simulink model "nasheq_model"  (R2023a)
settings: Solver=VariableStepAuto  StartTime=0.0  StopTime=6  RelTol=1e-3
values from neighbouring files (symbols this model uses):
  BESS2 =     [state_space.mat]    (also in state_space_and_controllers.mat)
  BESS3 =     [state_space.mat]    (also in state_space_and_controllers.mat)
  BESS6 =     [state_space.mat]    (also in state_space_and_controllers.mat)
  Grid =     [state_space.mat]    (also in state_space_and_controllers.mat)
  Load =     [state_space.mat]    (also in state_space_and_controllers.mat)
  PV1 =     [state_space.mat]    (also in state_space_and_controllers.mat)
  PV4 =     [state_space.mat]    (also in state_space_and_controllers.mat)
  PV5 =     [state_space.mat]    (also in state_space_and_controllers.mat)
  Ts = 0.0001    [cost_analysis.m]    (also in simulation_run.m)
libraries: slpidlib x6, spspowerguiLib x1
settings Model: Creator=paul  LastModifiedBy=paul
settings DataIOCC: Refine=4

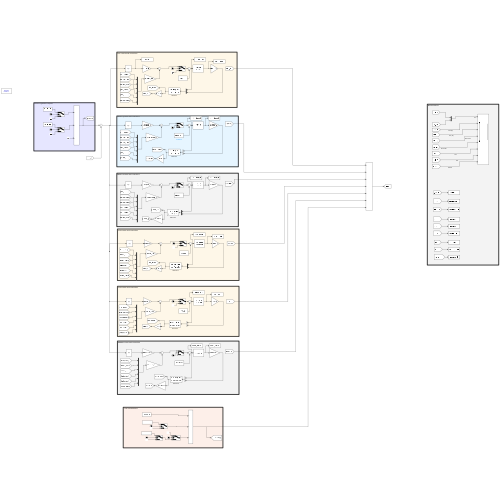
[thumbnail: Simulink's stored preview of the top-level diagram]
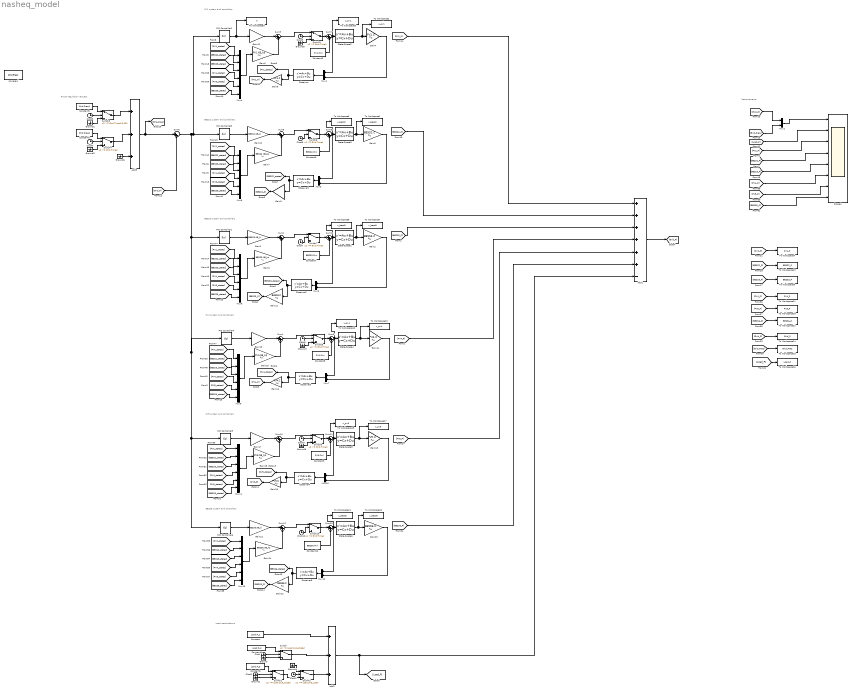
== system nasheq_model ==
  note: BESS2 system and controllers
  note: Measurements
  note: PV1 system and controllers
  note: Load perturbations
  note: Power regulation request
  note: BESS3 system and controllers
  note: PV4 system and controllers
  note: PV5 system and controllers
  note: BESS6 system and controllers
  Add1 : Sum  Inputs=++++++-
  Add2 : Sum  Inputs=+++
  Add3 : Sum  Inputs=+++
  Clock{,1..10} (11 alike) : Clock
  Constant : Constant  Value=Load.P_1
  Constant1 : Constant  Value=Load.P_2
  Constant10 : Constant  Value=BESS6.Pini
  Constant2 : Constant  Value=Load.P_3
  Constant3 : Constant  Value=Grid.Preq1
  Constant4 : Constant  Value=Grid.Preq2
  Constant5 : Constant  Value=PV1.Pini
  Constant6 : Constant  Value=BESS2.Pini
  Constant7 : Constant  Value=BESS3.Pini
  Constant8 : Constant  Value=PV4.Pini
  Constant9 : Constant  Value=PV5.Pini
  Gain1 : Gain  Gain=BESS3.NE_ki
  Gain10 : Gain  Gain=BESS2.NE_ki
  Gain11 : Gain  Gain=PV1.NE_ki
  Gain12 : Gain  Gain=BESS3.C  Multiplication=Matrix(K*u)
  Gain13 : Gain  Gain=PV4.NE_ki
  Gain14 : Gain  Gain=PV4.C  Multiplication=Matrix(K*u)
  Gain15 : Gain  Gain=PV4.NE_kp  Multiplication=Matrix(K*u)
  Gain16 : Gain  Gain=PV4.C  Multiplication=Matrix(K*u)
  Gain17 : Gain  Gain=PV5.NE_ki
  Gain18 : Gain  Gain=PV5.C  Multiplication=Matrix(K*u)
  Gain19 : Gain  Gain=PV5.NE_kp  Multiplication=Matrix(K*u)
  Gain2 : Gain  Gain=BESS3.C  Multiplication=Matrix(K*u)
  Gain20 : Gain  Gain=PV5.C  Multiplication=Matrix(K*u)
  Gain21 : Gain  Gain=BESS6.NE_ki
  Gain22 : Gain  Gain=BESS6.C  Multiplication=Matrix(K*u)
  Gain23 : Gain  Gain=BESS6.C  Multiplication=Matrix(K*u)
  Gain24 : Gain  Gain=BESS6.NE_kp  Multiplication=Matrix(K*u)
  Gain3 : Gain  Gain=BESS3.NE_kp  Multiplication=Matrix(K*u)
  Gain4 : Gain  Gain=PV1.C  Multiplication=Matrix(K*u)
  Gain5 : Gain  Gain=BESS2.C  Multiplication=Matrix(K*u)
  Gain6 : Gain  Gain=PV1.NE_kp  Multiplication=Matrix(K*u)
  Gain7 : Gain  Gain=BESS2.NE_kp  Multiplication=Matrix(K*u)
  Gain8 : Gain  Gain=PV1.C  Multiplication=Matrix(K*u)
  Gain9 : Gain  Gain=BESS2.C  Multiplication=Matrix(K*u)
  Ground{,1..8} (9 alike) : Ground
  Mux{1..3,6..7,10,12} (7 alike) : Mux  Inputs=2
  Mux{4..5,8..9,11,13} (6 alike) : Mux  Inputs=6
  Observer : StateSpace  A=PV1.kf_As  B=PV1.kf_Bs  C=PV1.kf_Cs  D=PV1.kf_Ds  InitialCondition=0
  Observer1 : StateSpace  A=BESS2.kf_As  B=BESS2.kf_Bs  C=BESS2.kf_Cs  D=BESS2.kf_Ds  InitialCondition=0
  Observer2 : StateSpace  A=BESS3.kf_As  B=BESS3.kf_Bs  C=BESS3.kf_Cs  D=BESS3.kf_Ds  InitialCondition=0
  Observer3 : StateSpace  A=PV4.kf_As  B=PV4.kf_Bs  C=PV4.kf_Cs  D=PV4.kf_Ds  InitialCondition=0
  Observer4 : StateSpace  A=PV5.kf_As  B=PV5.kf_Bs  C=PV5.kf_Cs  D=PV5.kf_Ds  InitialCondition=0
  Observer5 : StateSpace  A=BESS6.kf_As  B=BESS6.kf_Bs  C=BESS6.kf_Cs  D=BESS6.kf_Ds  InitialCondition=0
  PID Controller{1..6} (6 alike) : slpidlib/PID Controller  Controller=I  Form=Parallel  TimeDomain=Continuous-time  UseExternalTs=off  SampleTime=-1  IntegratorMethod=Forward Euler  FilterMethod=Forward Euler  ControllerParametersSource=internal  P=1  I=1  UseKiTs=off  D=0  N=100  UseFilter=on  TunerSelectOption=Transfer Function Based (PID Tuner App)  InitialConditionSource=internal  InitialConditionForIntegrator=0  InitialConditionForFilter=0  DifferentiatorICPrevScaledInput=0  ExternalReset=none  TrackingMode=off  Kt=1  LimitOutput=off  SatLimitsSource=internal  UpperSaturationLimit=inf  LowerSaturationLimit=-inf  LinearizeAsGain=on  AntiWindupMode=none  Kb=1  LimitIntegrator=off  UpperIntegratorSaturationLimit=inf  LowerIntegratorSaturationLimit=-inf  POutMin=[]  POutMax=[]  IOutMin=[]  IOutMax=[]  DOutMin=[]  DOutMax=[]  NOutMin=[]  NOutMax=[]  SumOutMin=[]  SumOutMax=[]  SaturationOutMin=[]  SaturationOutMax=[]  PParamMin=[]  PParamMax=[]  IParamMin=[]  IParamMax=[]  DParamMin=[]  DParamMax=[]  NParamMin=[]  NParamMax=[]  KbParamMin=[]  KbParamMax=[]  KtParamMin=[]  KtParamMax=[]  KbOutMin=[]  KbOutMax=[]  KtOutMin=[]  KtOutMax=[]  IntegratorOutMin=[]  IntegratorOutMax=[]  FilterOutMin=[]  FilterOutMax=[]  SumI1OutMin=[]  SumI1OutMax=[]  SumI2OutMin=[]  SumI2OutMax=[]  SumI3OutMin=[]  SumI3OutMax=[]  SumI4OutMin=[]  SumI4OutMax=[]  SumDOutMin=[]  SumDOutMax=[]  DifferentiatorOutMin=[]  DifferentiatorOutMax=[]  FilterDiffOutCoefMin=[]  FilterDiffOutCoefMax=[]  ReciprocalOutMin=[]  ReciprocalOutMax=[]  SumDenOutMin=[]  SumDenOutMax=[]  SumNumOutMin=[]  SumNumOutMax=[]  DivideOutMin=[]  DivideOutMax=[]  UdiffTsProdOutMin=[]  UdiffTsProdOutMax=[]  NTsProdOutMin=[]  NTsProdOutMax=[]  UintegralTsProdOutMin=[]  UintegralTsProdOutMax=[]  UngainTsProdOutMin=[]  UngainTsProdOutMax=[]  ClampingZeroOutDataTypeStr=Inherit: Inherit via back propagation  ClampingZeroOutMin=[]  ClampingZeroOutMax=[]  FilterDenConstantOutDataTypeStr=Inherit: Inherit via back propagation  FilterDenConstantOutMin=[]  FilterDenConstantOutMax=[]  PCopyOutDataTypeStr=Inherit: Inherit via back propagation  PCopyOutMin=[]  PCopyOutMax=[]  NCopyOutDataTypeStr=Inherit: Inherit via back propagation  NCopyOutMin=[]  NCopyOutMax=[]  IntegratorContinuousStateAttributes=''  IntegratorStateMustResolveToSignalObject=off  IntegratorRTWStateStorageClass=Auto  FilterContinuousStateAttributes=''  FilterStateMustResolveToSignalObject=off  FilterRTWStateStorageClass=Auto  ParallelPVariant=Disabled  IdealPVariant=Disabled  IVariant=InternalParameters  DVariant=Disabled  IntegratorVariant=Continuous  SatVariant=Disabled  AWVariant=Passthrough  PCopyVariant=Disabled  TRVariant=Disabled  FdbkBlocksVariant=Forward  IdealPFdbkVariant=Disabled  SatFdbkVariant=Disabled  DerivativeFilterVariant=Disabled  NVariant=Disabled  NCopyVariant=Disabled_SignalSpec  FilterICVariant=Disabled  IntegratorICVariant=InternalICs  ExternalResetVariant=Disabled  TRSumVariant=Passthrough  SumFdbkVariant=Disabled  SumVariant=Passthrough_I  TsampFilterVariant=InternalTs  TsampNgainVariant=Passthrough  TsampIntegralVariant=Disabled_SignalSpec  ExternalSaturationOutDataTypeStr=Inherit: Same as second input
  Scope1 : Scope  NumInputPorts=8
  State-Space1 : StateSpace  A=BESS3.A  B=BESS3.B  C=eye(2,2)  D=zeros(2,1)  InitialCondition=0
  State-Space2 : StateSpace  A=PV1.A  B=PV1.B  C=eye(2,2)  D=zeros(2,1)  InitialCondition=0
  State-Space3 : StateSpace  A=BESS2.A  B=BESS2.B  C=eye(2,2)  D=zeros(2,1)  InitialCondition=0
  State-Space4 : StateSpace  A=PV4.A  B=PV4.B  C=eye(2,2)  D=zeros(2,1)  InitialCondition=0
  State-Space5 : StateSpace  A=PV5.A  B=PV5.B  C=eye(2,2)  D=zeros(2,1)  InitialCondition=0
  State-Space6 : StateSpace  A=BESS6.A  B=BESS6.B  C=eye(2,2)  D=zeros(2,1)  InitialCondition=0
  Sum{1..5,7..13} (12 alike) : Sum  Inputs=|++
  Sum6 : Sum  Inputs=|+-
  Switch : Switch  Threshold=Load.sw2_closed  SaturateOnIntegerOverflow=off  InputSameDT=off
  Switch1 : Switch  Threshold=Load.sw3_closed  SaturateOnIntegerOverflow=off  InputSameDT=off
  Switch{5..10} (6 alike) : Switch  Threshold=Grid.Time1  SaturateOnIntegerOverflow=off  InputSameDT=off
  Switch2 : Switch  Threshold=Load.sw3_open  SaturateOnIntegerOverflow=off  InputSameDT=off
  Switch3 : Switch  Threshold=Grid.Time1-0.001  SaturateOnIntegerOverflow=off  InputSameDT=off
  Switch4 : Switch  Threshold=Grid.Time2  SaturateOnIntegerOverflow=off  InputSameDT=off
  To Workspace1 : ToWorkspace  VariableName=x_bess2  SaveFormat=Timeseries  SampleTime=Ts
  To Workspace10 : ToWorkspace  VariableName=x_pv4  SaveFormat=Timeseries  SampleTime=Ts
  To Workspace11 : ToWorkspace  VariableName=PV4_P  SaveFormat=Timeseries  SampleTime=Ts
  To Workspace12 : ToWorkspace  VariableName=u_pv4  SaveFormat=Timeseries  SampleTime=Ts
  To Workspace13 : ToWorkspace  VariableName=BESS2_P  SaveFormat=Timeseries  SampleTime=Ts
  To Workspace14 : ToWorkspace  VariableName=Grid_P  SaveFormat=Timeseries  SampleTime=Ts
  To Workspace15 : ToWorkspace  VariableName=Grid_Preq  SaveFormat=Timeseries  SampleTime=Ts
  To Workspace16 : ToWorkspace  VariableName=Load_P  SaveFormat=Timeseries  SampleTime=Ts
  To Workspace17 : ToWorkspace  VariableName=x_pv5  SaveFormat=Timeseries  SampleTime=Ts
  To Workspace18 : ToWorkspace  VariableName=PV5_P  SaveFormat=Timeseries  SampleTime=Ts
  To Workspace19 : ToWorkspace  VariableName=u_pv5  SaveFormat=Timeseries  SampleTime=Ts
  To Workspace2 : ToWorkspace  VariableName=x_pv1  SaveFormat=Timeseries  SampleTime=Ts
  To Workspace20 : ToWorkspace  VariableName=x_bess6  SaveFormat=Timeseries  SampleTime=Ts
  To Workspace21 : ToWorkspace  VariableName=u_bess6  SaveFormat=Timeseries  SampleTime=Ts
  To Workspace22 : ToWorkspace  VariableName=BESS6_P  SaveFormat=Timeseries  SampleTime=Ts
  To Workspace3 : ToWorkspace  VariableName=w  SaveFormat=Timeseries  SampleTime=Ts
  To Workspace4 : ToWorkspace  VariableName=PV1_P  SaveFormat=Timeseries  SampleTime=Ts
  To Workspace5 : ToWorkspace  VariableName=u_pv1  SaveFormat=Timeseries  SampleTime=Ts
  To Workspace6 : ToWorkspace  VariableName=u_bess2  SaveFormat=Timeseries  SampleTime=Ts
  To Workspace7 : ToWorkspace  VariableName=x_bess3  SaveFormat=Timeseries  SampleTime=Ts
  To Workspace8 : ToWorkspace  VariableName=u_bess3  SaveFormat=Timeseries  SampleTime=Ts
  To Workspace9 : ToWorkspace  VariableName=BESS3_P  SaveFormat=Timeseries  SampleTime=Ts
  powergui : spspowerguiLib/powergui  Priority=1  SimulationMode=Discrete  SampleTime=Ts  frequency=60  Iterations=50  frequencyindice=60  Pbase=100e6  ErrMax=1e-4  UnitsV=kV  UnitsW=MW  buscounter=0  FunctionMessages=off  echomessages=off  EnableUseOfTLC=off  CurrentSourceSwitches=off  DisableSnubberDevices=off  DisableRonSwitches=off  DisableVfSwitches=off  DisplayEquations=off  AutomaticDiscreteSolvers=off  SolverType=Tustin/Backward Euler (TBE)  Interpol=off  ExternalGateDelay=off  methode=off  Ts=100  x0status=blocks  SPID=on  SwTol=0  HookPort=off  NonlinearTolerance=1e-4  nMaxIteration=100  ContinueOnMaxIteration=off  RestoreLinks=warning  ResistiveCurrentMeasurement=off  Frange=[0:2:500]  Ylog=off  Xlog=on  ShowGrid=off  save=off  variable=ZData  structure=0  ZoomFFT=off  StartTime=0.0  cycles=1  DisplayStyle=1  fundamental=60  FreqAxis=off  MaxFrequency=1000  frequencyindicesteady=1  RmsSteady=1  display=off
  wires:
  Mux1/1 -> Observer/1
  Add1/1 -> [Grid_P]
  [BESS2_P] -> Scope1/4  "BESS2 (W)"
  Sum3/1 -> Switch5/1
  PID Controller3/1 -> Gain10/1
  Mux4/1 -> Gain6/1
  State-Space2/1 -> To Workspace2/1, Gain4/1
  Gain6/1 -> Sum3/2
  State-Space3/1 -> To Workspace1/1, Gain5/1
  Gain7/1 -> Sum5/2
  PID Controller2/1 -> To Workspace3/1, Gain11/1
  [PV1_P] -> Scope1/3  "PV1 (W)"
  Gain5/1 -> Mux3/2
  Mux3/1 -> Observer1/1
  Sum5/1 -> Switch6/1
  [PV1_states] -> Mux4/1
  Observer/1 -> Gain8/1, [PV1_states]
  [BESS2_states] -> Mux4/2
  Observer1/1 -> Gain9/1, [BESS2_states]
  Constant/1 -> Add2/1
  Constant1/1 -> Switch/1
  Clock/1 -> Switch/2
  Ground/1 -> Switch/3
  Switch/1 -> Add2/2
  [Load_P] -> Scope1/2  "Load (W)"
  [Grid_P] -> Sum6/2
  Ground1/1 -> Switch1/3
  Constant2/1 -> Switch1/1
  Clock1/1 -> Switch1/2
  Switch2/1 -> Add2/3
  Clock2/1 -> Switch2/2
  Switch1/1 -> Switch2/3
  Constant3/1 -> Switch3/1
  Clock3/1 -> Switch3/2
  Ground2/1 -> Switch3/3
  Switch3/1 -> Add3/1
  Add3/1 -> [Grid_Preq], Sum6/1
  Clock4/1 -> Switch4/2
  Constant4/1 -> Switch4/1
  Ground3/1 -> Switch4/3
  Switch4/1 -> Add3/2
  [Grid_P] -> Mux2/1
  Mux2/1 -> Scope1/1  "Grid"
  [Grid_Preq] -> Mux2/2
  Ground4/1 -> Switch2/1
  Constant5/1 -> Sum7/2
  Sum7/1 -> To Workspace5/1, Mux1/1, State-Space2/1
  Constant6/1 -> Sum8/2
  Sum8/1 -> Mux3/1, To Workspace6/1, State-Space3/1
  Switch5/1 -> Sum7/1
  Clock5/1 -> Switch5/2
  Switch6/1 -> Sum8/1
  Clock6/1 -> Switch6/2
  Ground5/1 -> Switch5/3
  Ground6/1 -> Add3/3
  Gain4/1 -> Mux1/2
  Add2/1 -> [Load_P], Add1/7
  Gain8/1 -> [PV1_P]
  [PV1_P] -> Add1/1
  Gain9/1 -> [BESS2_P]
  [BESS2_P] -> Add1/2
  Gain10/1 -> Sum5/1
  Gain11/1 -> Sum3/1
  [Grid_Preq] -> To Workspace15/1
  [Grid_P] -> To Workspace14/1
  [BESS2_P] -> To Workspace13/1
  [PV1_P] -> To Workspace4/1
  [Load_P] -> To Workspace16/1
  Sum2/1 -> Mux6/1, To Workspace8/1, State-Space1/1
  Gain3/1 -> Sum1/2
  Clock7/1 -> Switch7/2
  State-Space1/1 -> To Workspace7/1, Gain2/1
  Sum1/1 -> Switch7/1
  Constant7/1 -> Sum2/2
  Switch7/1 -> Sum2/1
  Gain2/1 -> Mux6/2
  Gain1/1 -> Sum1/1
  PID Controller1/1 -> Gain1/1
  Observer2/1 -> Gain12/1, [BESS3_states]
  [BESS3_P] -> Add1/3
  Mux6/1 -> Observer2/1
  Gain12/1 -> [BESS3_P]
  [BESS3_P] -> Scope1/5  "BESS3 (W)"
  [BESS3_P] -> To Workspace9/1
  [BESS3_states] -> Mux4/3
  Mux7/1 -> Observer3/1
  Ground7/1 -> Switch8/3
  Clock8/1 -> Switch8/2
  Sum4/1 -> Switch8/1
  Gain16/1 -> [PV4_P]
  [PV4_P] -> Add1/4
  Observer3/1 -> Gain16/1, [PV4_states]
  Sum9/1 -> To Workspace12/1, Mux7/1, State-Space4/1
  Switch8/1 -> Sum9/1
  Gain15/1 -> Sum4/2
  Gain13/1 -> Sum4/1
  Gain14/1 -> Mux7/2
  Constant8/1 -> Sum9/2
  State-Space4/1 -> To Workspace10/1, Gain14/1
  PID Controller4/1 -> Gain13/1
  Mux10/1 -> Observer4/1
  Ground8/1 -> Switch9/3
  Clock9/1 -> Switch9/2
  Sum10/1 -> Switch9/1
  Gain20/1 -> [PV5_P]
  [PV5_P] -> Add1/5
  Observer4/1 -> Gain20/1, [PV5_states]
  Sum11/1 -> To Workspace19/1, Mux10/1, State-Space5/1
  Switch9/1 -> Sum11/1
  Gain19/1 -> Sum10/2
  Gain17/1 -> Sum10/1
  Gain18/1 -> Mux10/2
  Constant9/1 -> Sum11/2
  State-Space5/1 -> To Workspace17/1, Gain18/1
  PID Controller5/1 -> Gain17/1
  Constant10/1 -> Sum13/2
  Gain22/1 -> [BESS6_P]
  Sum13/1 -> Mux12/1, To Workspace21/1, State-Space6/1
  Observer5/1 -> Gain22/1, [BESS6_states]
  Gain23/1 -> Mux12/2
  [BESS6_P] -> Add1/6
  Gain21/1 -> Sum12/1
  Clock10/1 -> Switch10/2
  Switch10/1 -> Sum13/1
  State-Space6/1 -> To Workspace20/1, Gain23/1
  Sum12/1 -> Switch10/1
  Sum6/1 -> PID Controller4/1, PID Controller6/1, PID Controller5/1, PID Controller1/1, PID Controller2/1, PID Controller3/1
  Gain24/1 -> Sum12/2
  PID Controller6/1 -> Gain21/1
  Mux12/1 -> Observer5/1
  [PV4_states] -> Mux4/4
  [PV5_states] -> Mux4/5
  [BESS6_states] -> Mux4/6
  [BESS6_states] -> Mux5/6
  [PV4_states] -> Mux5/4
  Mux5/1 -> Gain7/1
  [PV5_states] -> Mux5/5
  [BESS2_states] -> Mux5/2
  [BESS3_states] -> Mux5/3
  [PV1_states] -> Mux5/1
  [PV1_states] -> Mux8/1
  [BESS6_states] -> Mux8/6
  [BESS3_states] -> Mux8/3
  [PV5_states] -> Mux8/5
  [BESS2_states] -> Mux8/2
  [PV4_states] -> Mux8/4
  Mux8/1 -> Gain3/1
  [PV5_states] -> Mux9/5
  [PV4_states] -> Mux9/4
  Mux9/1 -> Gain15/1
  [BESS6_states] -> Mux9/6
  [BESS2_states] -> Mux9/2
  [PV1_states] -> Mux9/1
  [BESS3_states] -> Mux9/3
  [BESS3_states] -> Mux11/3
  [BESS6_states] -> Mux11/6
  [PV4_states] -> Mux11/4
  [PV5_states] -> Mux11/5
  [PV1_states] -> Mux11/1
  [BESS2_states] -> Mux11/2
  Mux11/1 -> Gain19/1
  [PV4_states] -> Mux13/4
  [BESS3_states] -> Mux13/3
  [BESS6_states] -> Mux13/6
  [PV1_states] -> Mux13/1
  [PV5_states] -> Mux13/5
  Mux13/1 -> Gain24/1
  [BESS2_states] -> Mux13/2
  [PV4_P] -> To Workspace11/1
  [PV5_P] -> To Workspace18/1
  [BESS6_P] -> To Workspace22/1
  [PV4_P] -> Scope1/6  "PV4"
  [PV5_P] -> Scope1/7  "PV5"
  [BESS6_P] -> Scope1/8  "BESS6"
